simulink model "AccelerometerDemo4LRLs"  (R2022b)
settings: Solver=FixedStepAuto  StartTime=0.0  StopTime=1000  FixedStep=1e-2  RelTol=1e-3  EnableMultiTasking=on
libraries: frdmk64flib x1, dsparch4 x1, dspstat3 x1
settings Model: ExtModeTrigDuration=5  Creator=Admin  LastModifiedBy=Admin
settings OptimizationCC: EnhancedBackFolding=on  PassReuseOutputArgsAs=Individual arguments  ZeroExternalMemoryAtStartup=off  ZeroInternalMemoryAtStartup=off  MaxStackSize=64  OptimizeBlockOrder=speed  DifferentSizesBufferReuse=on  OptimizationCustomize=off  EfficientTunableParamExpr=on
settings DebuggingCC: ParameterTunabilityLossMsg=error
settings HardwareCC: ProdBitPerPointer=32  ProdBitPerSizeT=32  ProdBitPerPtrDiffT=32  ProdLargestAtomicInteger=Long  ProdLargestAtomicFloat=Double  ProdWordSize=32  ProdHWDeviceType=ARM Compatible->ARM Cortex
settings SFSimCC: MATLABDynamicMemAlloc=off
settings RTWCC: Description=Embedded Coder  SystemTargetFile=ert.tlc  HardwareBoard=NXP FRDM-K64F  TLCOptions="-aInlineSetEventsForThisBaseRateFcn=TLC_FALSE -aSuppressMultiTaskScheduler=TLC_FALSE  -aRateBasedStepFcn=0"  TemplateMakefile=ert_default_tmf  Toolchain=GNU Tools for ARM Embedded Processors
settings CodeAppCC: ForceParamTrailComments=on  IgnoreCustomStorageClasses=off  OperatorAnnotations=on  SimulinkDataObjDesc=on  SFDataObjDesc=on  InsertBlockDesc=on
settings ERTTargetCC: ExtModeTransport=4  ExtModeMexFile=sendToCommService

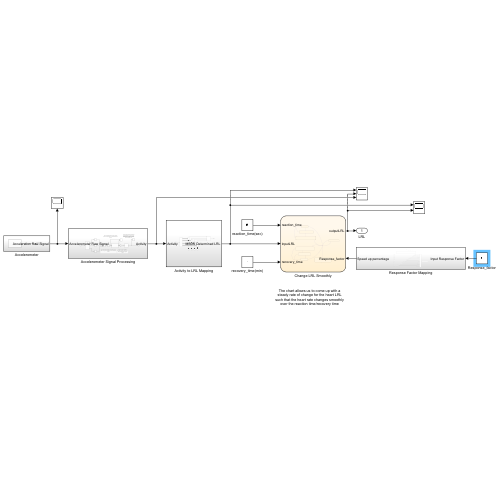
[thumbnail: Simulink's stored preview of the top-level diagram]
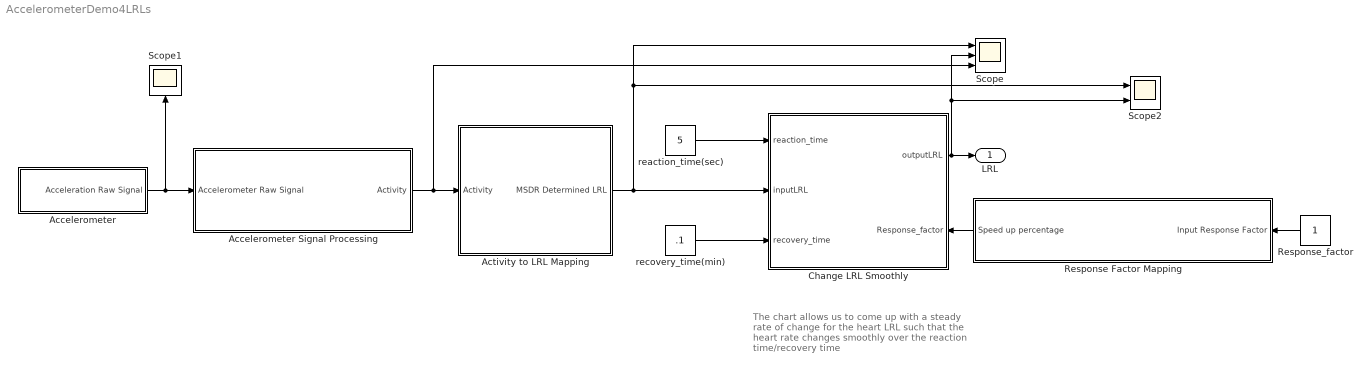
== system AccelerometerDemo4LRLs ==
  note: The chart allows us to come up with a steady rate of change for the heart LRL such that the heart rate changes smoothly over the reaction time/recovery time
  Accelerometer : Subsystem
  Accelerometer Signal Processing : Subsystem
  Activity to LRL Mapping : Subsystem
  Change LRL Smoothly : Stateflow chart  TreatAsAtomicUnit=on
      settings: PortSchema="{\"entries\":[{\"content\":{\"sides\":[{\"content\":{\"connectorIds\":[\"In3\",\"In2\",\"In4\"]},\"type\":\"ConnectorPlacement.EquallySpacedRectSide\",\"uuid\":\"85af1beb-61ae-4766-b408-8225321ec4a4\"},{\"content\":{\"connectorIds\":[\"Out1\",\"In1\"],\"side\":\"RIGHT\"},\"type\":\"ConnectorPlacement.EquallySpacedRectSide\",\"uuid\":\"bdf3d147-5894-49ca-bdec-54ebdf64bfa8\"},{\"content\":{\"connectorIds\":[],\"side\":\"TOP\"},\"type\":\"ConnectorPlacement.EquallySpacedRectSide\",\"uuid\":\"42bc5e47-54de-4fed-b1f0-fe2ea6e0cd28\"},{\"content\":{\"connectorIds\":[],\"side\":\"BOTTOM\"},\"type\":\"ConnectorPlacement.EquallySpacedRectSide\",\"uuid\":\"092d377f-872f-4731-90ca-5dcd29f87b08\"}]},\"type\":\"ConnectorPlacement.EquallySpacedConnector\",\"uuid\":\"a2c4c5d6-6aa5-4141-8747-f931ac594277\"}],\"packageUris\":[\"http://schema.mathworks.com/mf0/Connector/R2020b\"],\"version\":\"1.0\"}"
  Response Factor Mapping : Subsystem
  Response_factor : Constant
  Scope : Scope  NumInputPorts=3
  Scope1 : Scope
  Scope2 : Scope  NumInputPorts=2
  reaction_time(sec) : Constant  Value=5
  recovery_time(min) : Constant  Value=.1
  LRL : Outport
  wires:
  Accelerometer Signal Processing/1(Activity) -> Activity to LRL Mapping/1(Activity), Scope/3
  Accelerometer/1(Acceleration Raw Signal) -> Accelerometer Signal Processing/1(Accelerometer Raw Signal), Scope1/1
  recovery_time(min)/1 -> Change LRL Smoothly/4(recovery_time)
  Response_factor/1 -> Response Factor Mapping/1(Input Response Factor)
  Activity to LRL Mapping/1(MSDR Determined LRL) -> Change LRL Smoothly/2(inputLRL), Scope2/1, Scope/1
  reaction_time(sec)/1 -> Change LRL Smoothly/3(reaction_time)
  Response Factor Mapping/1(Speed up percentage) -> Change LRL Smoothly/1(Response_factor)
  Change LRL Smoothly/1(outputLRL) -> LRL/1, Scope/2, Scope2/2

== system AccelerometerDemo4LRLs/Accelerometer ==
  FXOS8700 6-Axes Sensor : frdmk64flib/FXOS8700 6-Axes Sensor  Activesensor=Accelerometer only  ODR=800Hz  HybridODR=400Hz  Accelfullrange=-8g to +8g  SampleTime=-1
  Acceleration Raw Signal : Outport
  wires:
  FXOS8700 6-Axes Sensor/1 -> Acceleration Raw Signal/1

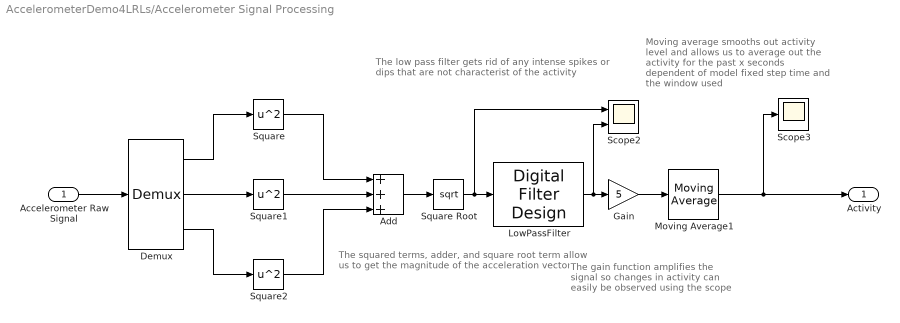
== system AccelerometerDemo4LRLs/Accelerometer Signal Processing ==
  note: The squared terms, adder, and square root term allow us to get the magnitude of the acceleration vector
  note: Moving average smooths out activity level and allows us to average out the activity for the past x seconds dependent of model fixed step time and the window used
  note: The gain function amplifies the signal so changes in activity can easily be observed using the scope
  note: The low pass filter gets rid of any intense spikes or dips that are not characterist of the activity
  Accelerometer Raw Signal : Inport
  Add : Sum  Inputs=+++
  Demux : Demux  Outputs=3
      settings: DisplayOption=none
  Gain : Gain  Gain=5
  LowPassFilter : dsparch4/Digital Filter Design  mwdsp_browser_bugfix_var=off
  Moving Average1 : dspstat3/Moving Average  Method=Sliding window  ForgettingFactorPort=off  SpecifyWindowLength=on  WindowLength=500  OverlapLength=499  AllowArbitraryInputLength=off  ForgettingFactor=0.9  SimulateUsing=Code generation
  Scope2 : Scope  NumInputPorts=2
  Scope3 : Scope
  Square : Math  Operator=square
  Square Root : Sqrt
  Square1 : Math  Operator=square
  Square2 : Math  Operator=square
  Activity : Outport
  wires:
  LowPassFilter/1 -> Scope2/2, Gain/1
  Gain/1 -> Moving Average1/1
  Square2/1 -> Add/3
  Demux/1 -> Square/1
  Square1/1 -> Add/2
  Square Root/1 -> Scope2/1, LowPassFilter/1
  Moving Average1/1 -> Activity/1, Scope3/1
  Demux/3 -> Square2/1
  Add/1 -> Square Root/1
  Demux/2 -> Square1/1
  Square/1 -> Add/1
  Accelerometer Raw Signal/1 -> Demux/1

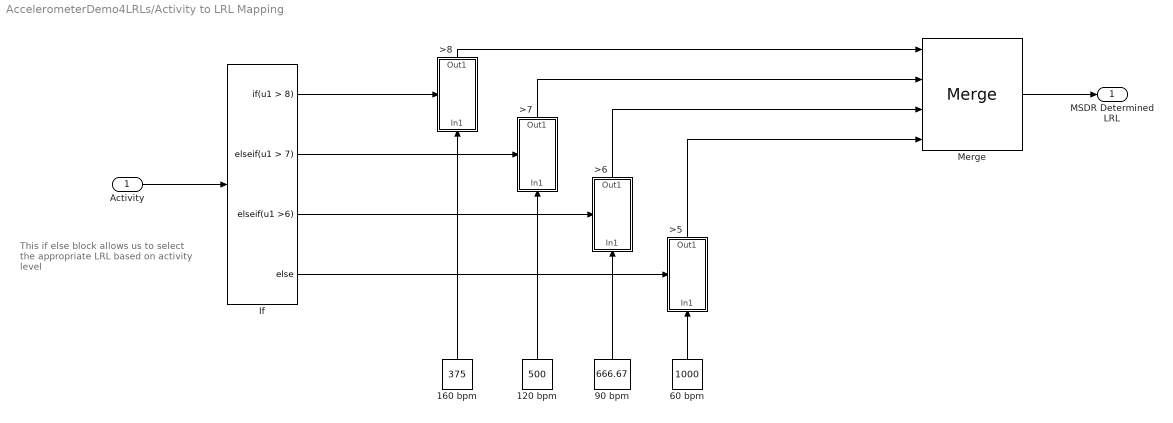
== system AccelerometerDemo4LRLs/Activity to LRL Mapping ==
  note: This if else block allows us to select the appropriate LRL based on activity level
  Activity : Inport
  120 bpm : Constant  Value=500
  160 bpm : Constant  Value=375
  60 bpm : Constant  Value=1000
  90 bpm : Constant  Value=666.67
  >5 : Subsystem  TreatAsAtomicUnit=on
  >6 : Subsystem  TreatAsAtomicUnit=on
  >7 : Subsystem  TreatAsAtomicUnit=on
  >8 : Subsystem  TreatAsAtomicUnit=on
  If : If  IfExpression=u1 > 8  ElseIfExpressions=u1 > 7, u1 >6
  Merge : Merge  Inputs=4
  MSDR Determined LRL : Outport
  wires:
  60 bpm/1 -> >5/1(In1)
  Merge/1 -> MSDR Determined LRL/1
  Activity/1 -> If/1
  If/1 -> >8/Action
  If/2 -> >7/Action
  If/3 -> >6/Action
  If/4 -> >5/Action
  160 bpm/1 -> >8/1(In1)
  120 bpm/1 -> >7/1(In1)
  90 bpm/1 -> >6/1(In1)
  >8/1(Out1) -> Merge/1
  >7/1(Out1) -> Merge/2
  >6/1(Out1) -> Merge/3
  >5/1(Out1) -> Merge/4

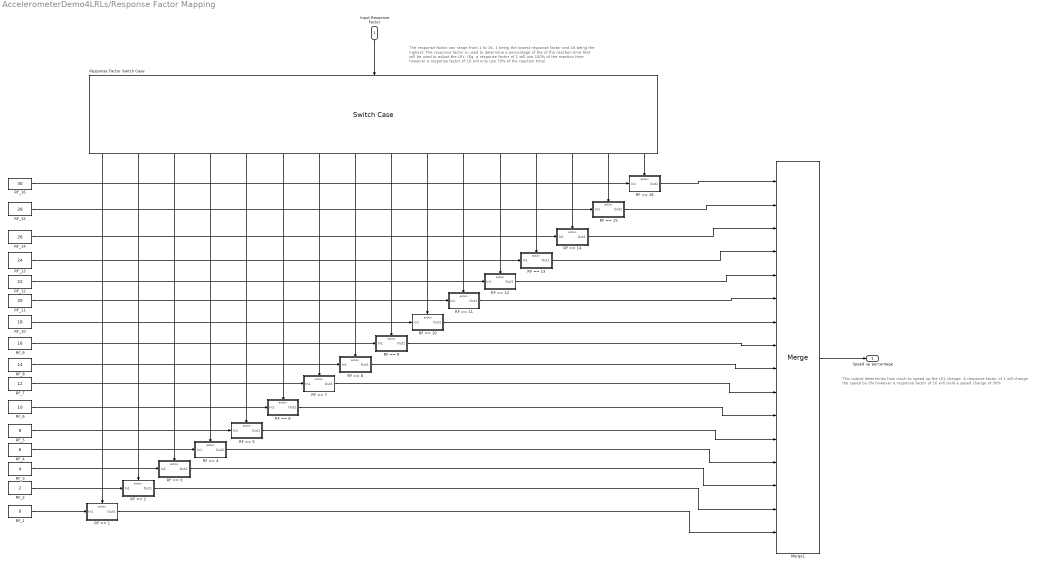
== system AccelerometerDemo4LRLs/Response Factor Mapping ==
  note: This output determines how much to speed up the LRL change. A response factor of 1 will change the speed by 0% however a response factor of 16 will yield a speed change of 30%
  note: The response factor can range from 1 to 16. 1 being the lowest response factor and 16 being the highest.
      | The response factor is used to determine a percentage of the of the reaction time that will be used to adjust the LRL. (Eg, a response factor of 1 will use 100% of the reaction time however a response factor of 16 will only use 70% of the reaction time)
  Input Response Factor : Inport
  Merge1 : Merge  Inputs=16
  RF == 1 : Subsystem  TreatAsAtomicUnit=on
  RF == 10 : Subsystem  TreatAsAtomicUnit=on
  RF == 11 : Subsystem  TreatAsAtomicUnit=on
  RF == 12 : Subsystem  TreatAsAtomicUnit=on
  RF == 13 : Subsystem  TreatAsAtomicUnit=on
  RF == 14 : Subsystem  TreatAsAtomicUnit=on
  RF == 15 : Subsystem  TreatAsAtomicUnit=on
  RF == 16 : Subsystem  TreatAsAtomicUnit=on
  RF == 2 : Subsystem  TreatAsAtomicUnit=on
  RF == 3 : Subsystem  TreatAsAtomicUnit=on
  RF == 4 : Subsystem  TreatAsAtomicUnit=on
  RF == 5 : Subsystem  TreatAsAtomicUnit=on
  RF == 6 : Subsystem  TreatAsAtomicUnit=on
  RF == 7 : Subsystem  TreatAsAtomicUnit=on
  RF == 8 : Subsystem  TreatAsAtomicUnit=on
  RF == 9 : Subsystem  TreatAsAtomicUnit=on
  RF_1 : Constant  Value=0
  RF_10 : Constant  Value=18
  RF_11 : Constant  Value=20
  RF_12 : Constant  Value=22
  RF_13 : Constant  Value=24
  RF_14 : Constant  Value=26
  RF_15 : Constant  Value=28
  RF_16 : Constant  Value=30
  RF_2 : Constant  Value=2  OutDataTypeStr=double
  RF_3 : Constant  Value=4
  RF_4 : Constant  Value=6
  RF_5 : Constant  Value=8
  RF_6 : Constant  Value=10
  RF_7 : Constant  Value=12
  RF_8 : Constant  Value=14
  RF_9 : Constant  Value=16
  Response Factor Switch Case : SwitchCase  CaseConditions={1,2,3,4,5,6,7,8,9,10,11,12,13,14,15,16}  ShowDefaultCase=off
  Speed up percentage : Outport
  wires:
  Input Response Factor/1 -> Response Factor Switch Case/1
  RF == 1/1(Out1) -> Merge1/16
  RF == 5/1(Out1) -> Merge1/12
  RF_8/1 -> RF == 8/1(In1)
  RF_9/1 -> RF == 9/1(In1)
  RF_2/1 -> RF == 2/1(In1)
  Response Factor Switch Case/5 -> RF == 5/Action
  Response Factor Switch Case/16 -> RF == 16/Action
  Response Factor Switch Case/6 -> RF == 6/Action
  RF_10/1 -> RF == 10/1(In1)
  Response Factor Switch Case/1 -> RF == 1/Action
  RF == 16/1(Out1) -> Merge1/1
  RF == 4/1(Out1) -> Merge1/13
  Response Factor Switch Case/3 -> RF == 3/Action
  RF == 9/1(Out1) -> Merge1/8
  Response Factor Switch Case/9 -> RF == 9/Action
  RF == 13/1(Out1) -> Merge1/4
  RF == 14/1(Out1) -> Merge1/3
  Response Factor Switch Case/2 -> RF == 2/Action
  RF_1/1 -> RF == 1/1(In1)
  Response Factor Switch Case/10 -> RF == 10/Action
  RF == 6/1(Out1) -> Merge1/11
  RF == 15/1(Out1) -> Merge1/2
  RF_13/1 -> RF == 13/1(In1)
  RF_16/1 -> RF == 16/1(In1)
  RF == 7/1(Out1) -> Merge1/10
  RF_5/1 -> RF == 5/1(In1)
  RF_7/1 -> RF == 7/1(In1)
  RF_4/1 -> RF == 4/1(In1)
  RF == 3/1(Out1) -> Merge1/14
  Response Factor Switch Case/12 -> RF == 12/Action
  Response Factor Switch Case/14 -> RF == 14/Action
  Response Factor Switch Case/4 -> RF == 4/Action
  RF_3/1 -> RF == 3/1(In1)
  RF == 12/1(Out1) -> Merge1/5
  Response Factor Switch Case/8 -> RF == 8/Action
  RF_15/1 -> RF == 15/1(In1)
  RF == 8/1(Out1) -> Merge1/9
  Response Factor Switch Case/7 -> RF == 7/Action
  Response Factor Switch Case/11 -> RF == 11/Action
  Response Factor Switch Case/15 -> RF == 15/Action
  RF_6/1 -> RF == 6/1(In1)
  Merge1/1 -> Speed up percentage/1
  RF_12/1 -> RF == 12/1(In1)
  RF == 11/1(Out1) -> Merge1/6
  RF_11/1 -> RF == 11/1(In1)
  Response Factor Switch Case/13 -> RF == 13/Action
  RF == 2/1(Out1) -> Merge1/15
  RF_14/1 -> RF == 14/1(In1)
  RF == 10/1(Out1) -> Merge1/7

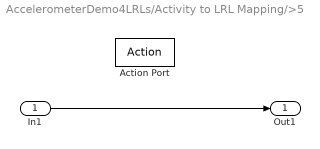
== system AccelerometerDemo4LRLs/Activity to LRL Mapping/>5 ==
  In1 : Inport
  Action Port : ActionPort  ActionPortLabel=else
  Out1 : Outport
  wires:
  In1/1 -> Out1/1

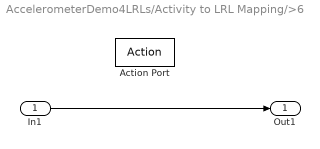
== system AccelerometerDemo4LRLs/Activity to LRL Mapping/>6 ==
  In1 : Inport
  Action Port : ActionPort  ActionPortLabel=elseif( u1 >6)
  Out1 : Outport
  wires:
  In1/1 -> Out1/1

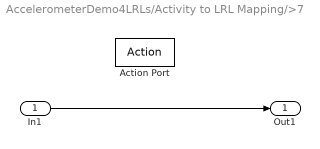
== system AccelerometerDemo4LRLs/Activity to LRL Mapping/>7 ==
  In1 : Inport
  Action Port : ActionPort  ActionPortLabel=elseif(u1 > 7)
  Out1 : Outport
  wires:
  In1/1 -> Out1/1

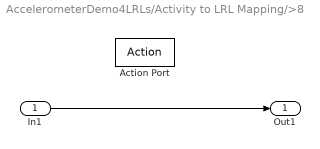
== system AccelerometerDemo4LRLs/Activity to LRL Mapping/>8 ==
  In1 : Inport
  Action Port : ActionPort  ActionPortLabel=if(u1 > 8)
  Out1 : Outport
  wires:
  In1/1 -> Out1/1

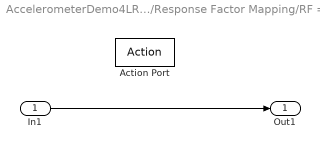
== system AccelerometerDemo4LRLs/Response Factor Mapping/RF == 1 ==
  In1 : Inport
  Action Port : ActionPort  ActionPortLabel=case [ 1 ]:
  Out1 : Outport
  wires:
  In1/1 -> Out1/1

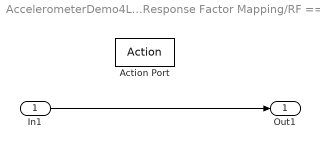
== system AccelerometerDemo4LRLs/Response Factor Mapping/RF == 10 ==
  In1 : Inport
  Action Port : ActionPort  ActionPortLabel=case [ 10 ]:
  Out1 : Outport
  wires:
  In1/1 -> Out1/1

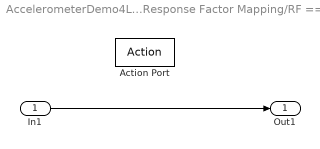
== system AccelerometerDemo4LRLs/Response Factor Mapping/RF == 11 ==
  In1 : Inport
  Action Port : ActionPort  ActionPortLabel=case [ 11 ]:
  Out1 : Outport
  wires:
  In1/1 -> Out1/1

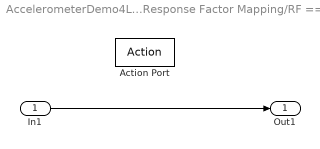
== system AccelerometerDemo4LRLs/Response Factor Mapping/RF == 12 ==
  In1 : Inport
  Action Port : ActionPort  ActionPortLabel=case [ 12 ]:
  Out1 : Outport
  wires:
  In1/1 -> Out1/1

== system AccelerometerDemo4LRLs/Response Factor Mapping/RF == 13 ==
  In1 : Inport
  Action Port : ActionPort  ActionPortLabel=case [ 13 ]:
  Out1 : Outport
  wires:
  In1/1 -> Out1/1

== system AccelerometerDemo4LRLs/Response Factor Mapping/RF == 14 ==
  In1 : Inport
  Action Port : ActionPort  ActionPortLabel=case [ 14 ]:
  Out1 : Outport
  wires:
  In1/1 -> Out1/1

== system AccelerometerDemo4LRLs/Response Factor Mapping/RF == 15 ==
  In1 : Inport
  Action Port : ActionPort  ActionPortLabel=case [ 15 ]:
  Out1 : Outport
  wires:
  In1/1 -> Out1/1

== system AccelerometerDemo4LRLs/Response Factor Mapping/RF == 16 ==
  In1 : Inport
  Action Port : ActionPort  ActionPortLabel=case [ 16 ]:
  Out1 : Outport
  wires:
  In1/1 -> Out1/1

== system AccelerometerDemo4LRLs/Response Factor Mapping/RF == 2 ==
  In1 : Inport
  Action Port : ActionPort  ActionPortLabel=case [ 2 ]:
  Out1 : Outport
  wires:
  In1/1 -> Out1/1

== system AccelerometerDemo4LRLs/Response Factor Mapping/RF == 3 ==
  In1 : Inport
  Action Port : ActionPort  ActionPortLabel=case [ 3 ]:
  Out1 : Outport
  wires:
  In1/1 -> Out1/1

== system AccelerometerDemo4LRLs/Response Factor Mapping/RF == 4 ==
  In1 : Inport
  Action Port : ActionPort  ActionPortLabel=case [ 4 ]:
  Out1 : Outport
  wires:
  In1/1 -> Out1/1

== system AccelerometerDemo4LRLs/Response Factor Mapping/RF == 5 ==
  In1 : Inport
  Action Port : ActionPort  ActionPortLabel=case [ 5 ]:
  Out1 : Outport
  wires:
  In1/1 -> Out1/1

== system AccelerometerDemo4LRLs/Response Factor Mapping/RF == 6 ==
  In1 : Inport
  Action Port : ActionPort  ActionPortLabel=case [ 6 ]:
  Out1 : Outport
  wires:
  In1/1 -> Out1/1

== system AccelerometerDemo4LRLs/Response Factor Mapping/RF == 7 ==
  In1 : Inport
  Action Port : ActionPort  ActionPortLabel=case [ 7 ]:
  Out1 : Outport
  wires:
  In1/1 -> Out1/1

== system AccelerometerDemo4LRLs/Response Factor Mapping/RF == 8 ==
  In1 : Inport
  Action Port : ActionPort  ActionPortLabel=case [ 8 ]:
  Out1 : Outport
  wires:
  In1/1 -> Out1/1

== system AccelerometerDemo4LRLs/Response Factor Mapping/RF == 9 ==
  In1 : Inport
  Action Port : ActionPort  ActionPortLabel=case [ 9 ]:
  Out1 : Outport
  wires:
  In1/1 -> Out1/1

== stateflow chart AccelerometerDemo4LRLs/Change LRL Smoothly ==
  state Raise_HeartRate
    entry:
    outputLRL = currLRL
  state Increment_currLRL_Down
    entry:
    currLRL = currLRL - rate_of_change
  state Speed_Up_HeartRate
    entry:
    rate_of_change = (outputLRL-inputLRL)/(reaction_time*10) *(1+(Response_factor/100))
    %Says how many seconds I need to decrease the LRL per tenth of a second passed in the simulation
    currLRL = outputLRL %setting the step change LRL to its starting point
    setPoint = inputLRL
  state Wait_For_Change
    entry:
    outputLRL = inputLRL;
  state Slow_Down_HeartRate
    entry:
    rate_of_change = (inputLRL - outputLRL)/(recovery_time*60*10) *(1+(Response_factor/100))
    %how many seconds to increase the LRL by for each tenth of a second passed in the simulation
    %reaction time is in minutes
    currLRL = outputLRL
    setPoint = inputLRL
  state Increment_currLRL_Up
    entry:
    currLRL = currLRL + rate_of_change
  state Start_Here
    entry:
    outputLRL = 1000 %no LRL has been set to the heart yet so we'll start off at 60 bpm
  state Lower_HeartRate
    entry:
    outputLRL = currLRL
  Raise_HeartRate -> (junction 54) [order 2] : [outputLRL > inputLRL]
  Raise_HeartRate -> (junction 51) [order 1] : [outputLRL <= inputLRL]
  (junction 54) -> Increment_currLRL_Down [order 2] : [setPoint == inputLRL]
  (junction 54) -> Speed_Up_HeartRate [order 1] : [setPoint ~= inputLRL]
  Increment_currLRL_Down -> Raise_HeartRate : after(100,msec)
  Speed_Up_HeartRate -> Increment_currLRL_Down
  (junction 51) -> Speed_Up_HeartRate [order 1] : [outputLRL>inputLRL]
  (junction 51) -> Wait_For_Change [order 2] : [outputLRL <= inputLRL+0.1 && outputLRL >= inputLRL-0.1]
  Wait_For_Change -> (junction 51)
  (junction 51) -> Slow_Down_HeartRate [order 3] : [outputLRL<inputLRL]
  Lower_HeartRate -> (junction 51) [order 1] : [outputLRL >= inputLRL]
  Start_Here -> (junction 51)
  (junction 64) -> Slow_Down_HeartRate [order 2] : [setPoint ~= inputLRL]
  Slow_Down_HeartRate -> Increment_currLRL_Up
  (junction 64) -> Increment_currLRL_Up [order 1] : [setPoint == inputLRL]
  Increment_currLRL_Up -> Lower_HeartRate : after(100,msec)
  Lower_HeartRate -> (junction 64) [order 2] : [outputLRL < inputLRL]
  (default) -> Start_Here
  data: Response_factor input; inputLRL input; reaction_time input; recovery_time input; currLRL local; outputLRL output; rate_of_change local; setPoint local
